simulink model "SimpleAnimation"  (R2023b)
settings: Solver=VariableStepAuto  StartTime=0.0  StopTime=10.0  RelTol=1e-3
libraries: vrlib x2
settings Model: Creator=BeanieBabyJ  LastModifiedBy=BeanieBabyJ

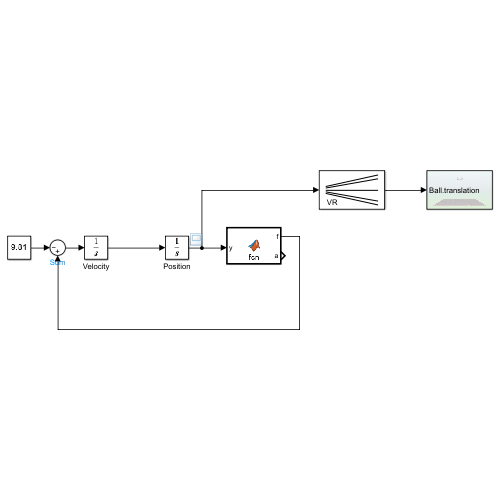
[thumbnail: Simulink's stored preview of the top-level diagram]
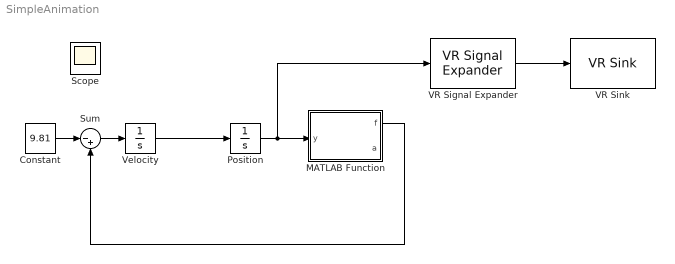
== system SimpleAnimation ==
  Constant : Constant  Value=9.81
  MATLAB Function : MATLAB Function  TreatAsAtomicUnit=on
  Position : Integrator  InitialCondition=20
  Sum : Sum  Inputs=|-+
  VR Signal Expander : vrlib/VR Signal Expander  outwidth=3  outidx=[2]
  VR Sink : vrlib/VR Sink  InstantiateOnLoad=on  SampleTime=0.1  ViewEnable=on  RemoteChange=off  RemoteView=off  FieldsWritten=Ball.translation.3.1.1.double  WorldFileName=SimpleAnimationWorld.slx.x3d  AutoView=off  VideoDimensions=[]  AllowVariableSize=off
  Velocity : Integrator
  Scope : Scope
  wires:
  Velocity/1 -> Position/1
  Position/1 -> VR Signal Expander/1, MATLAB Function/1(y)
  Constant/1 -> Sum/1
  Sum/1 -> Velocity/1
  MATLAB Function/1(f) -> Sum/2
  VR Signal Expander/1 -> VR Sink/1

== matlab function SimpleAnimation/MATLAB Function ==
  data: y input; f output; a output
function [f,a] = fcn(y)

if y <= 1e-4
    y = 1e-4;
end

if y<1.5
    f=500*(1.5-y);
    a=sqrt(1.5^3/y);
else
    f=0;
    a=1.5;
end
